simulink model "Q3_t"  (R2021b)
settings: Solver=VariableStepAuto  StartTime=0.0  StopTime=15  RelTol=1e-3
settings Model: Creator=nima8  LastModifiedBy=nima8

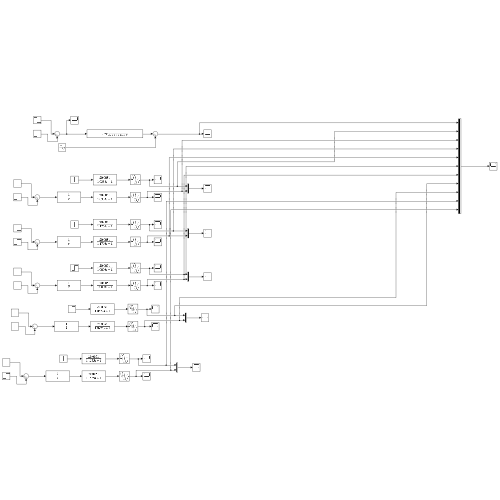
[thumbnail: Simulink's stored preview of the top-level diagram]
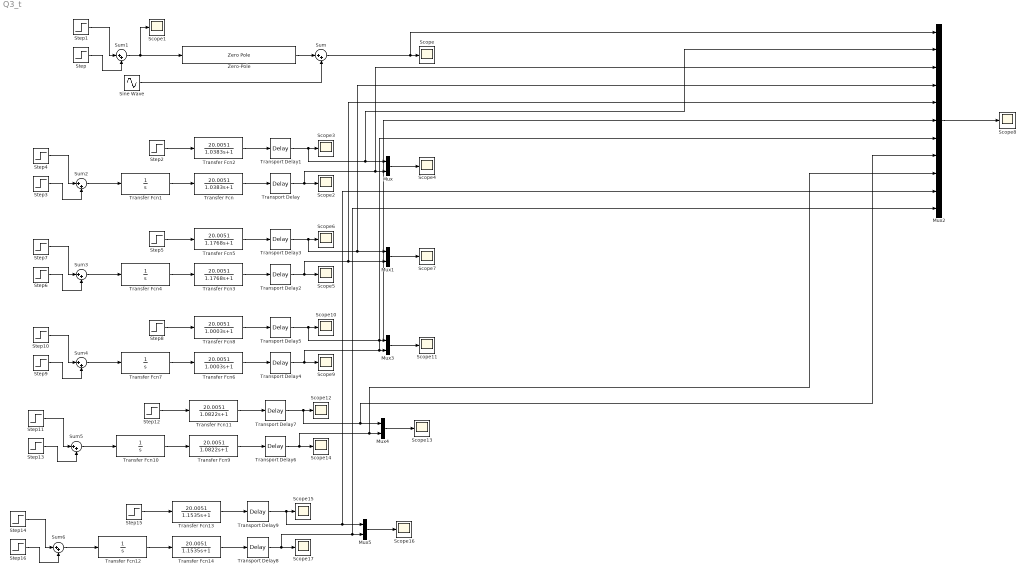
== system Q3_t ==
  Mux{,1,3..5} (5 alike) : Mux  Inputs=2
  Mux2 : Mux  Inputs=11
  Scope{,1..17} (18 alike) : Scope
  Sine Wave : Sin  Amplitude=0.05  Frequency=40  SampleTime=0
  Step{,3,6,9,13,16} (6 alike) : Step  Time=0  After=0  SampleTime=0
  Step{1,4,7,10..11,14} (6 alike) : Step  Time=0.1  Before=1  After=0  SampleTime=0
  Step{2,5,8,12,15} (5 alike) : Step  Time=0  After=0.1  SampleTime=0
  Sum{,1..6} (7 alike) : Sum  Inputs=|++
  Transfer Fcn : TransferFcn  Numerator=[20.0051]  Denominator=[1.0383 1]
  Transfer Fcn{1,4,7,10,12} (5 alike) : TransferFcn  Denominator=[1 0]
  Transfer Fcn11 : TransferFcn  Numerator=[20.0051]  Denominator=[1.0822 1]
  Transfer Fcn13 : TransferFcn  Numerator=[20.0051]  Denominator=[1.1535 1]
  Transfer Fcn14 : TransferFcn  Numerator=[20.0051]  Denominator=[1.1535 1]
  Transfer Fcn2 : TransferFcn  Numerator=[20.0051]  Denominator=[1.0383 1]
  Transfer Fcn3 : TransferFcn  Numerator=[20.0051]  Denominator=[1.1768 1]
  Transfer Fcn5 : TransferFcn  Numerator=[20.0051]  Denominator=[1.1768 1]
  Transfer Fcn6 : TransferFcn  Numerator=[20.0051]  Denominator=[1.0003 1]
  Transfer Fcn8 : TransferFcn  Numerator=[20.0051]  Denominator=[1.0003 1]
  Transfer Fcn9 : TransferFcn  Numerator=[20.0051]  Denominator=[1.0822 1]
  Transport Delay{,1..9} (10 alike) : TransportDelay  DelayTime=0.8488
  Zero-Pole : ZeroPole  Zeros=[]  Poles=[ 0 -1 -2 -3]  Gain=[120]
  wires:
  Zero-Pole/1 -> Sum/1
  Sum/1 -> Mux2/1, Scope/1
  Sine Wave/1 -> Sum/2
  Step1/1 -> Sum1/1
  Step/1 -> Sum1/2
  Sum1/1 -> Zero-Pole/1, Scope1/1
  Transfer Fcn/1 -> Transport Delay/1
  Transfer Fcn1/1 -> Transfer Fcn/1
  Transport Delay/1 -> Mux2/3, Mux/2, Scope2/1
  Transport Delay1/1 -> Mux2/2, Mux/1, Scope3/1
  Transfer Fcn2/1 -> Transport Delay1/1
  Step2/1 -> Transfer Fcn2/1
  Step4/1 -> Sum2/1
  Step3/1 -> Sum2/2
  Sum2/1 -> Transfer Fcn1/1
  Mux/1 -> Scope4/1
  Mux1/1 -> Scope7/1
  Transfer Fcn5/1 -> Transport Delay3/1
  Step5/1 -> Transfer Fcn5/1
  Transport Delay2/1 -> Mux2/5, Mux1/2, Scope5/1
  Transport Delay3/1 -> Mux2/4, Mux1/1, Scope6/1
  Transfer Fcn4/1 -> Transfer Fcn3/1
  Step6/1 -> Sum3/2
  Step7/1 -> Sum3/1
  Sum3/1 -> Transfer Fcn4/1
  Transfer Fcn3/1 -> Transport Delay2/1
  Mux2/1 -> Scope8/1
  Mux3/1 -> Scope11/1
  Transfer Fcn8/1 -> Transport Delay5/1
  Step8/1 -> Transfer Fcn8/1
  Transport Delay4/1 -> Mux2/7, Mux3/2, Scope9/1
  Transport Delay5/1 -> Mux3/1, Mux2/6, Scope10/1
  Transfer Fcn7/1 -> Transfer Fcn6/1
  Step9/1 -> Sum4/2
  Step10/1 -> Sum4/1
  Sum4/1 -> Transfer Fcn7/1
  Transfer Fcn6/1 -> Transport Delay4/1
  Step11/1 -> Sum5/1
  Sum5/1 -> Transfer Fcn10/1
  Transfer Fcn9/1 -> Transport Delay6/1
  Transport Delay7/1 -> Mux2/8, Mux4/1, Scope12/1
  Transport Delay6/1 -> Mux2/9, Mux4/2, Scope14/1
  Step12/1 -> Transfer Fcn11/1
  Mux4/1 -> Scope13/1
  Transfer Fcn11/1 -> Transport Delay7/1
  Step13/1 -> Sum5/2
  Transfer Fcn10/1 -> Transfer Fcn9/1
  Sum6/1 -> Transfer Fcn12/1
  Step14/1 -> Sum6/1
  Transfer Fcn12/1 -> Transfer Fcn14/1
  Transport Delay8/1 -> Mux2/11, Mux5/2, Scope17/1
  Transfer Fcn13/1 -> Transport Delay9/1
  Transfer Fcn14/1 -> Transport Delay8/1
  Step16/1 -> Sum6/2
  Step15/1 -> Transfer Fcn13/1
  Mux5/1 -> Scope16/1
  Transport Delay9/1 -> Mux2/10, Mux5/1, Scope15/1
